simulink model "sampleModel1641_5_sub_sub"  (R2023a)
settings: Solver=VariableStepAuto  StartTime=0.0  StopTime=10.0  RelTol=1e-3
libraries: hdlsllib x4, simulink x1
settings Model: Creator=user1  LastModifiedBy=user1
settings OptimizationCC: BlockReduction=off  ConditionallyExecuteInputs=off

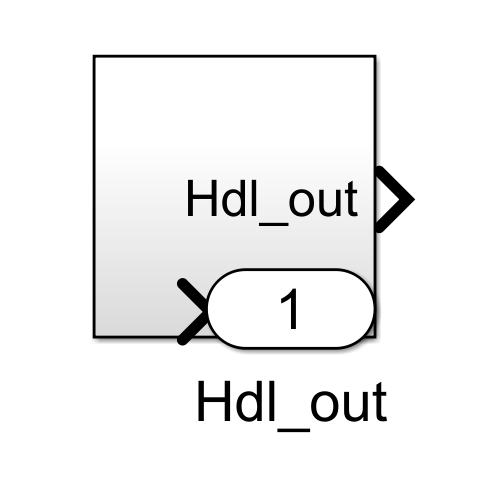
[thumbnail: Simulink's stored preview of the top-level diagram]
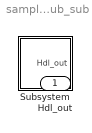
== system sampleModel1641_5_sub_sub ==
  Subsystem : Subsystem
  Hdl_out : Outport  OutDataTypeStr=uint8

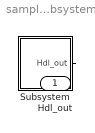
== system sampleModel1641_5_sub_sub/Subsystem ==
  Subsystem : Subsystem
  Hdl_out : Outport  OutDataTypeStr=uint8
  wires:
  Subsystem/1(Hdl_out) -> Hdl_out/1

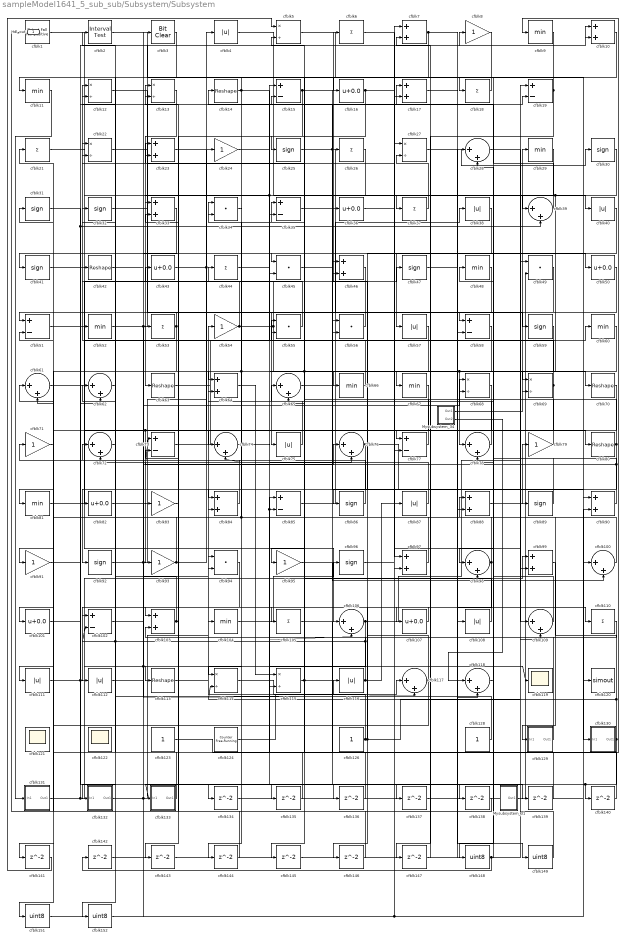
== system sampleModel1641_5_sub_sub/Subsystem/Subsystem ==
  Mysubsystem_31 : Subsystem  TreatAsAtomicUnit=on  RTWFcnName=Mysubsystem_31
      settings: RTWFcnNameOpts=User specified  RTWFileNameOpts=Use function name
  Mysubsystem_34 : Subsystem  TreatAsAtomicUnit=on  RTWFcnName=Mysubsystem_34
      settings: RTWFcnNameOpts=User specified  RTWFileNameOpts=Use function name
  cfblk1 : hdlsllib/Logic and Bit Operations/Detect Fall Nonpositive  vinit=0  OutDataTypeStr=uint8
  cfblk{7,10,17,23,33,46,64,84,88,90,97,99,103} (13 alike) : Sum  OutDataTypeStr=uint8
  cfblk{28,39,61..62,65,72,74,76,78,98,100,106,109,117..118} (15 alike) : Sum  Inputs=|++  OutDataTypeStr=uint8
  cfblk{16,36,43,50,82,101,107} (7 alike) : Bias  Bias=0.0  SaturateOnIntegerOverflow=off
  cfblk{15,19,35,51,58,73,77,85,102} (9 alike) : Sum  Inputs=+-  OutDataTypeStr=uint8
  cfblk{9,11,29,48,52,60,66..67,81,104} (10 alike) : MinMax  OutDataTypeStr=uint8
  cfblk{6,18,21,26,37,44,53,105,110} (9 alike) : Sum  Inputs=+  OutDataTypeStr=uint8
  cfblk{4,38,40,57,75,87,108,111..112,116} (10 alike) : Abs  OutDataTypeStr=uint8  SaturateOnIntegerOverflow=off
  cfblk{14,42,63,70,80,113} (6 alike) : Reshape
  cfblk{5,12..13,22,27,68..69,114..115} (9 alike) : Product  Inputs=*/  OutDataTypeStr=uint8  RndMeth=Zero  SaturateOnIntegerOverflow=on
  cfblk119 : Scope
  cfblk120 : ToWorkspace  VariableName=simout  SaveFormat=Timeseries  SampleTime=-1
  cfblk121 : Scope
      settings: Floating=on
  cfblk122 : Scope
      settings: Floating=on
  cfblk123 : Constant  OutDataTypeStr=uint8  SampleTime=-1
  cfblk124 : hdlsllib/Sources/Counter Free-Running  NumBits=16  tsamp=-1
  cfblk126 : Constant  OutDataTypeStr=uint8  SampleTime=-1
  cfblk128 : Constant  OutDataTypeStr=uint8  SampleTime=-1
  cfblk129 : Subsystem
      settings: LibrarySourceBlock=|
      | hdlsllib/Ports &
      | Subsystems/Subsystem
  cfblk130 : Subsystem
      settings: LibrarySourceBlock=|
      | hdlsllib/Ports &
      | Subsystems/Subsystem
  cfblk131 : Subsystem
      settings: LibrarySourceBlock=|
      | hdlsllib/Ports &
      | Subsystems/Subsystem
  cfblk132 : Subsystem
      settings: LibrarySourceBlock=|
      | hdlsllib/Ports &
      | Subsystems/Subsystem
  cfblk133 : Subsystem
      settings: LibrarySourceBlock=|
      | hdlsllib/Ports &
      | Subsystems/Subsystem
  cfblk{134..147} (14 alike) : Delay  SampleTime=1
  cfblk{148..149,151..152} (4 alike) : DataTypeConversion  OutDataTypeStr=uint8  SaturateOnIntegerOverflow=off  RndMeth=Floor
  cfblk2 : hdlsllib/Logic and Bit Operations/Interval Test  IntervalClosedRight=on  uplimit=0.5  IntervalClosedLeft=on  lowlimit=-0.5  OutDataTypeStr=uint8
  cfblk{8,24,54,71,79,83,91,93,95} (9 alike) : Gain  OutDataTypeStr=uint8
  cfblk{25,30..32,41,47,59,86,89,92,96} (11 alike) : Signum
  cfblk3 : simulink/Logic and Bit Operations/Bit Clear  iBit=0
      settings: LibrarySourceBlock=|
      | hdlsllib/Logic and Bit
      | Operations/Bit Clear
  cfblk{34,45,49,55..56,94} (6 alike) : DotProduct  OutDataTypeStr=uint8
  Hdl_out : Outport  OutDataTypeStr=uint8
  wires:
  Mysubsystem_34/2(Out2) -> cfblk118/1
  Mysubsystem_34/1(Out1) -> cfblk69/2
  Mysubsystem_31/1(Out1) -> cfblk49/2
  cfblk152/1 -> cfblk120/1, cfblk97/2
  cfblk151/1 -> cfblk3/1
  cfblk149/1 -> cfblk49/1
  cfblk47/1 -> cfblk149/1
  cfblk148/1 -> cfblk142/1, cfblk48/1
  cfblk147/1 -> cfblk7/2
  cfblk70/1 -> cfblk147/1
  cfblk146/1 -> cfblk61/2
  cfblk145/1 -> cfblk98/2
  cfblk144/1 -> cfblk23/2
  cfblk143/1 -> cfblk27/1
  cfblk142/1 -> cfblk109/2
  cfblk141/1 -> cfblk5/1
  cfblk71/1 -> cfblk141/1
  cfblk140/1 -> cfblk65/2
  cfblk139/1 -> cfblk51/2
  cfblk17/1 -> cfblk139/1
  cfblk138/1 -> cfblk1/1
  cfblk105/1 -> cfblk138/1
  cfblk137/1 -> cfblk28/1
  cfblk31/1 -> cfblk137/1
  cfblk136/1 -> cfblk56/1
  cfblk44/1 -> cfblk136/1
  cfblk135/1 -> cfblk85/1
  cfblk91/1 -> cfblk135/1
  cfblk134/1 -> cfblk90/2
  cfblk34/1 -> cfblk134/1
  cfblk5/1 -> cfblk130/1(In1)
  cfblk74/1 -> cfblk76/2, cfblk144/1
  cfblk101/1 -> cfblk62/2
  cfblk133/1(Out1) -> cfblk22/1
  cfblk78/1 -> cfblk64/2
  cfblk24/1 -> cfblk67/1
  cfblk33/1 -> cfblk41/1
  cfblk26/1 -> cfblk64/1, cfblk45/2
  cfblk14/1 -> cfblk85/2, cfblk106/2, cfblk114/1
  cfblk8/1 -> cfblk74/1
  cfblk35/1 -> cfblk40/1
  cfblk115/1 -> cfblk19/2, cfblk5/2
  cfblk110/1 -> cfblk103/2
  cfblk128/1 -> cfblk62/1
  cfblk63/1 -> cfblk36/1
  cfblk124/1 -> cfblk116/1
  cfblk54/1 -> cfblk26/1, cfblk118/2, cfblk33/2
  cfblk15/1 -> cfblk33/1, cfblk70/1
  cfblk87/1 -> cfblk72/2
  cfblk43/1 -> cfblk50/1, cfblk77/2
  cfblk72/1 -> cfblk32/1
  cfblk32/1 -> cfblk17/2
  cfblk42/1 -> cfblk45/1
  cfblk3/1 -> cfblk152/1
  cfblk57/1 -> cfblk91/1
  cfblk68/1 -> cfblk83/1, cfblk81/1
  cfblk118/1 -> cfblk88/1
  cfblk109/1 -> cfblk65/1
  cfblk61/1 -> cfblk4/1
  cfblk62/1 -> cfblk12/2
  cfblk67/1 -> cfblk95/1
  cfblk6/1 -> cfblk99/2
  cfblk89/1 -> cfblk68/1
  cfblk83/1 -> cfblk43/1
  cfblk94/1 -> cfblk112/1
  cfblk86/1 -> cfblk61/1
  cfblk77/1 -> cfblk34/2
  cfblk65/1 -> cfblk56/2
  cfblk95/1 -> cfblk100/2
  cfblk129/1(Out1) -> cfblk23/1
  cfblk90/1 -> cfblk28/2, cfblk73/1
  cfblk48/1 -> cfblk66/1
  cfblk114/1 -> cfblk117/1
  cfblk99/1 -> cfblk129/1(In1)
  cfblk104/1 -> cfblk96/1
  cfblk10/1 -> cfblk78/2
  cfblk66/1 -> cfblk42/1
  cfblk50/1 -> cfblk82/1
  cfblk56/1 -> cfblk53/1
  cfblk40/1 -> cfblk86/1
  cfblk29/1 -> cfblk107/1
  cfblk75/1 -> cfblk44/1
  cfblk18/1 -> cfblk11/1
  cfblk82/1 -> cfblk93/1
  cfblk2/1 -> cfblk18/1
  cfblk69/1 -> cfblk98/1, cfblk55/1
  cfblk55/1 -> cfblk12/1
  cfblk60/1 -> cfblk132/1(In1)
  cfblk93/1 -> cfblk47/1, cfblk21/1
  cfblk49/1 -> cfblk148/1
  cfblk112/1 -> cfblk119/1, cfblk76/1
  cfblk37/1 -> cfblk27/2
  cfblk7/1 -> cfblk25/1, cfblk110/1
  cfblk28/1 -> cfblk109/1
  cfblk73/1 -> cfblk15/1
  cfblk106/1 -> cfblk19/1, cfblk115/2
  cfblk111/1 -> cfblk39/2, cfblk15/2, cfblk113/1
  cfblk23/1 -> cfblk59/1
  cfblk16/1 -> cfblk97/1, cfblk105/1
  cfblk131/1(Out1) -> cfblk99/1, cfblk6/1
  cfblk92/1 -> cfblk24/1, cfblk68/2
  cfblk130/1(Out1) -> cfblk133/1(In1), cfblk140/1, cfblk114/2, cfblk84/2
  cfblk21/1 -> cfblk35/2
  cfblk76/1 -> cfblk100/1, cfblk84/1
  cfblk13/1 -> cfblk63/1
  cfblk9/1 -> cfblk58/2
  cfblk39/1 -> cfblk14/1
  cfblk19/1 -> cfblk16/1, cfblk77/1
  cfblk117/1 -> cfblk46/1, cfblk151/1
  cfblk108/1 -> cfblk35/1
  cfblk98/1 -> cfblk2/1, cfblk146/1
  cfblk12/1 -> cfblk58/1
  cfblk100/1 -> cfblk34/1, cfblk13/1
  cfblk22/1 -> cfblk17/1
  cfblk46/1 -> cfblk75/1
  cfblk25/1 -> cfblk108/1, cfblk88/2
  cfblk1/1 -> cfblk90/1
  cfblk103/1 -> cfblk72/1, cfblk73/2
  cfblk36/1 -> cfblk39/1
  cfblk79/1 -> cfblk29/1
  cfblk59/1 -> cfblk101/1, cfblk145/1
  cfblk27/1 -> cfblk30/1
  cfblk102/1 -> cfblk94/2
  cfblk30/1 -> cfblk69/1, cfblk143/1
  cfblk84/1 -> cfblk71/1
  cfblk88/1 -> cfblk79/1
  cfblk51/1 -> cfblk80/1
  cfblk97/1 -> cfblk31/1
  cfblk58/1 -> cfblk74/2, cfblk102/1, cfblk78/1
  cfblk4/1 -> cfblk37/1
  cfblk41/1 -> cfblk106/1
  cfblk132/1(Out1) -> cfblk104/1, cfblk55/2
  cfblk96/1 -> cfblk7/1
  cfblk80/1 -> cfblk92/1, cfblk22/2
  cfblk52/1 -> cfblk8/1, cfblk117/2, cfblk10/2
  cfblk123/1 -> cfblk9/1
  cfblk81/1 -> cfblk60/1
  cfblk113/1 -> cfblk94/1
  cfblk45/1 -> cfblk10/1
  cfblk107/1 -> cfblk103/1
  cfblk116/1 -> cfblk52/1, cfblk102/2, cfblk13/2, cfblk87/1
  cfblk11/1 -> cfblk131/1(In1)
  cfblk64/1 -> cfblk115/1
  cfblk38/1 -> cfblk57/1
  cfblk85/1 -> cfblk38/1
  cfblk53/1 -> cfblk51/1, cfblk111/1
  cfblk126/1 -> cfblk89/1, cfblk46/2, cfblk54/1

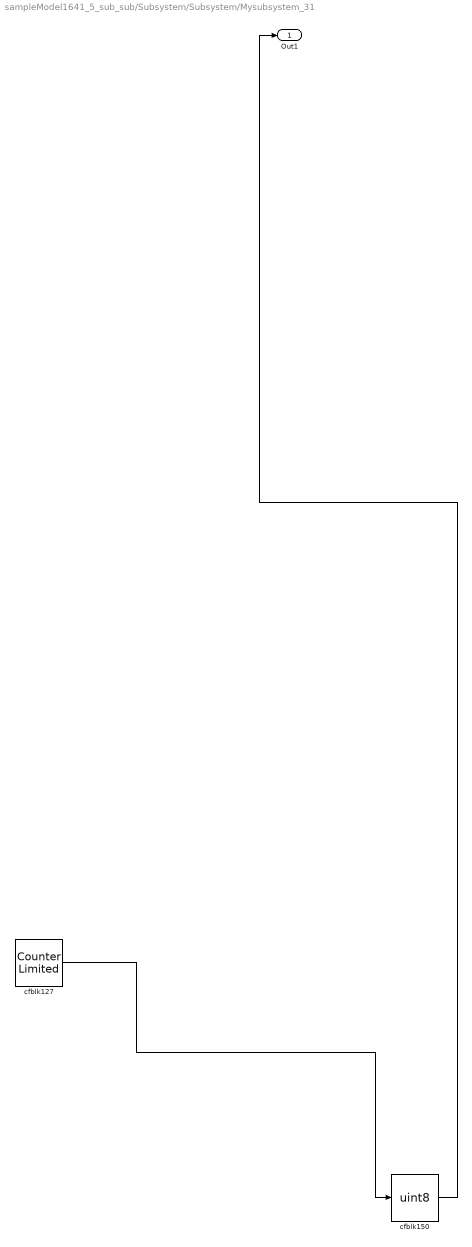
== system sampleModel1641_5_sub_sub/Subsystem/Subsystem/Mysubsystem_31 ==
  cfblk127 : hdlsllib/Sources/Counter Limited  uplimit=7  tsamp=-1
  cfblk150 : DataTypeConversion  OutDataTypeStr=uint8  SaturateOnIntegerOverflow=off  RndMeth=Floor
  Out1 : Outport
  wires:
  cfblk127/1 -> cfblk150/1
  cfblk150/1 -> Out1/1

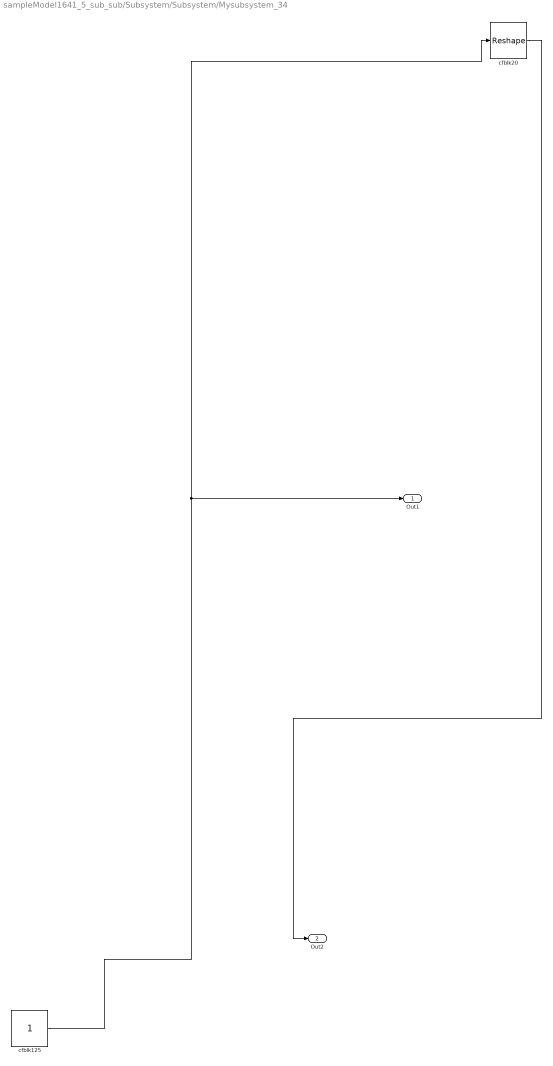
== system sampleModel1641_5_sub_sub/Subsystem/Subsystem/Mysubsystem_34 ==
  cfblk125 : Constant  SampleTime=-1
  cfblk20 : Reshape
  Out1 : Outport
  Out2 : Outport  Port=2
  wires:
  cfblk125/1 -> Out1/1, cfblk20/1
  cfblk20/1 -> Out2/1

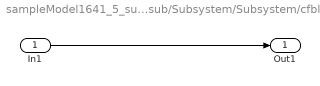
== system sampleModel1641_5_sub_sub/Subsystem/Subsystem/cfblk129 ==
  In1 : Inport
  Out1 : Outport
  wires:
  In1/1 -> Out1/1

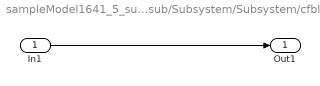
== system sampleModel1641_5_sub_sub/Subsystem/Subsystem/cfblk130 ==
  In1 : Inport
  Out1 : Outport
  wires:
  In1/1 -> Out1/1

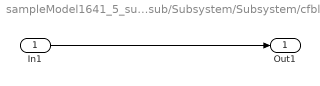
== system sampleModel1641_5_sub_sub/Subsystem/Subsystem/cfblk131 ==
  In1 : Inport
  Out1 : Outport
  wires:
  In1/1 -> Out1/1

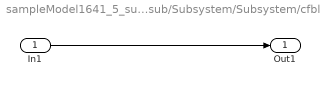
== system sampleModel1641_5_sub_sub/Subsystem/Subsystem/cfblk132 ==
  In1 : Inport
  Out1 : Outport
  wires:
  In1/1 -> Out1/1

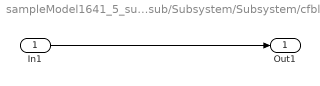
== system sampleModel1641_5_sub_sub/Subsystem/Subsystem/cfblk133 ==
  In1 : Inport
  Out1 : Outport
  wires:
  In1/1 -> Out1/1
